simulink model "chap10_5sim"  (Simulink 3.00)
settings: Solver=ode45  StartTime=0.0  StopTime=3  FixedStep=0.001  RelTol=1e-3
settings Model: LastModifiedBy=liu

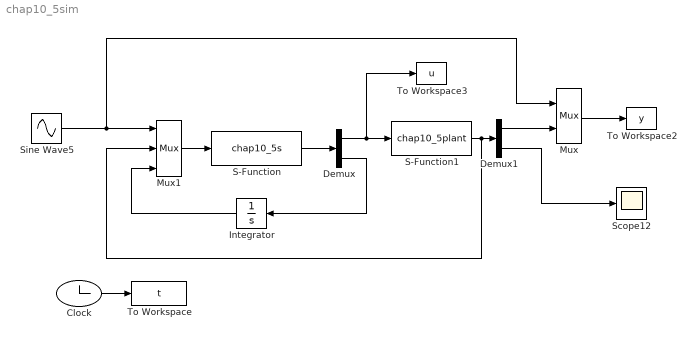
== system chap10_5sim ==
  Clock : Clock
  Demux : Demux  Outputs=2
  Demux1 : Demux  Outputs=2
  Integrator : Integrator  Orientation=left  ExternalReset=none  InitialConditionSource=internal  InitialCondition=0  LimitOutput=off  UpperSaturationLimit=inf  LowerSaturationLimit=-inf  ShowSaturationPort=off  ShowStatePort=off  AbsoluteTolerance=auto
  Mux : Mux  Inputs=2
      settings: DisplayOption=none
  Mux1 : Mux  Inputs=3
      settings: DisplayOption=none
  S-Function : S-Function  FunctionName=chap10_5s  PortCounts=[]  SFunctionModules=''
  S-Function1 : S-Function  FunctionName=chap10_5plant  PortCounts=[]  SFunctionModules=''
  Scope12 : Scope
      settings: TickLabels=on  TimeRange=3  YMin=-3.5  YMax=3.5  SaveToWorkspace=off  SaveName=ScopeData  MaxRows=50000
  Sine Wave5 : Sin  Amplitude=0.50  Frequency=1*2*pi  Phase=0  SampleTime=0
  To Workspace : ToWorkspace  VariableName=t  SampleTime=-1  SaveFormat=Matrix
  To Workspace2 : ToWorkspace  VariableName=y  SampleTime=-1  SaveFormat=Matrix
  To Workspace3 : ToWorkspace  VariableName=u  SampleTime=-1  SaveFormat=Matrix
  wires:
  Mux1/1 -> S-Function/1
  S-Function/1 -> Demux/1
  Clock/1 -> To Workspace/1
  Integrator/1 -> Mux1/3
  Demux/2 -> Integrator/1
  Mux/1 -> To Workspace2/1
  Demux1/1 -> Mux/2
  S-Function1/1 -> Demux1/1, Mux1/2
  Demux1/2 -> Scope12/1
  Demux/1 -> S-Function1/1, To Workspace3/1
  Sine Wave5/1 -> Mux1/1, Mux/1
